simulink model "RLC"  (R2024a)
settings: Solver=VariableStepAuto  StartTime=0.0  StopTime=0.5  RelTol=1e-3
model workspace (MAT data in the model file):
  C = 0.001
  L = 10
  R = 400
settings Model: Creator=hp  LastModifiedBy=NB
settings SolverCC: AlgebraicLoopSolver=TrustRegion
settings DataIOCC: ReturnWorkspaceOutputs=off
settings DebuggingCC: UnconnectedInputMsg=warning  UnconnectedOutputMsg=warning  UnconnectedLineMsg=warning  ArithmeticOperatorsInVariantConditions=warning
settings ModelReferenceCC: EnableRefExpFcnMdlSchedulingChecks=on
settings SFSimCC: CustomCodeUndefinedFunction=UseInterfaceOnly
settings RTWCC: GPUComputeCapability=3.5

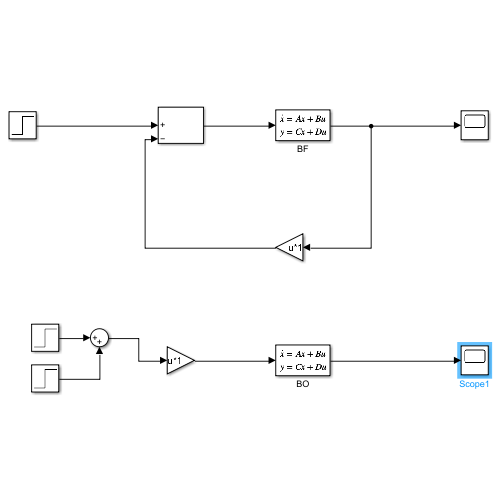
[thumbnail: Simulink's stored preview of the top-level diagram]
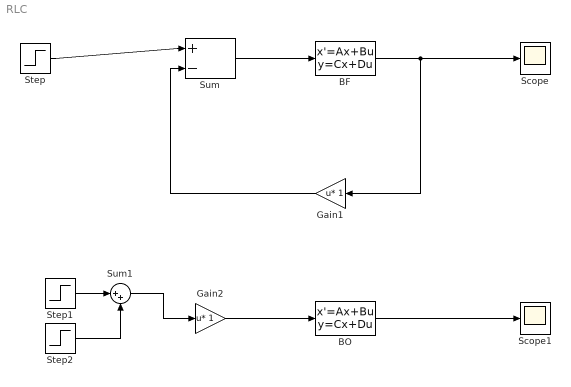
== system RLC ==
  BF : StateSpace  A=[-R/L 0 -1/L; 1 0 0; 1/C 0 0]  B=[1/L; 0; 0]  C=[0 0 1]  D=0  InitialCondition=0
  BO : StateSpace  A=[-R/L 0 -1/L; 1 0 0; 1/C 0 0]  B=[1/L; 0; 0]  C=[0 0 1]  D=0  InitialCondition=0
  Gain1 : Gain  Multiplication=Matrix(u*K)
  Gain2 : Gain  Multiplication=Matrix(u*K)
  Scope : Scope
  Scope1 : Scope
  Step : Step  Time=0  SampleTime=0
  Step1 : Step  Time=0  SampleTime=0
  Step2 : Step  Time=0.001  SampleTime=0
  Sum : Sum  Inputs=|+-
  Sum1 : Sum  Inputs=|++
  wires:
  Sum/1 -> BF/1
  BF/1 -> Gain1/1, Scope/1
  Gain1/1 -> Sum/2
  Gain2/1 -> BO/1
  BO/1 -> Scope1/1
  Step/1 -> Sum/1
  Sum1/1 -> Gain2/1
  Step1/1 -> Sum1/1
  Step2/1 -> Sum1/2
